simulink model "arduino"  (R2015b)
settings: Solver=VariableStepAuto  StartTime=0.0  StopTime=100.0  RelTol=1e-3
undefined symbols (not defined in the file or in its folder): serial
libraries: instrumentlib x3
settings Model: Creator=ovi  LastModifiedBy=ovi

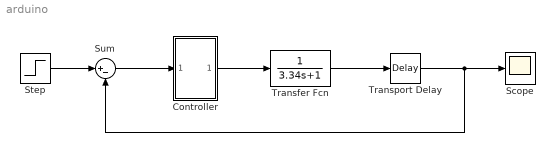
== system arduino ==
  "Controller " : Subsystem
  Scope : Scope
  Step : Step  SampleTime=0
  Sum : Sum  Inputs=|+-
  Transfer Fcn : TransferFcn  Denominator=[3.34 1]
  Transport Delay : TransportDelay  DelayTime=1.86
  wires:
  Sum/1 -> "Controller "/1(In1)
  "Controller "/1(Out1) -> Transfer Fcn/1
  Transfer Fcn/1 -> Transport Delay/1
  Transport Delay/1 -> Sum/2, Scope/1
  Step/1 -> Sum/1

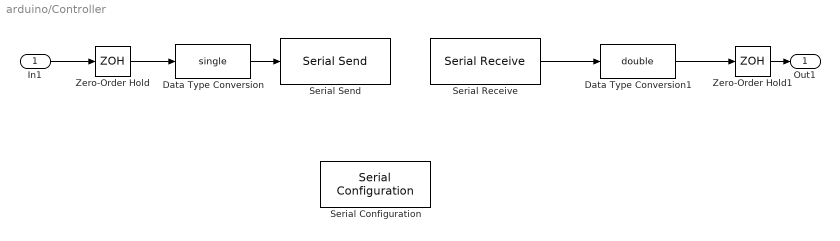
== system arduino/Controller  ==
  In1 : Inport
  Data Type Conversion : DataTypeConversion  OutDataTypeStr=single
  Data Type Conversion1 : DataTypeConversion  OutDataTypeStr=double
  Serial Configuration : instrumentlib/Serial Configuration  Priority=-200000  ComPortMenu=/dev/cu.usbmodem14101  ComPort=/dev/cu.usbmodem14101  ObjConstructor=serial('/dev/cu.usbmodem14101');  BaudRate=9600  DataBits=8  Parity=none  StopBits=1  FlowControl=none  Timeout=10  ByteOrder=LittleEndian
  Serial Receive : instrumentlib/Serial Receive  ComPortMenu=/dev/cu.usbmodem14101  ComPort=/dev/cu.usbmodem14101  ObjConstructor=serial('/dev/cu.usbmodem14101');  Terminator=<none>  DataSize=[1 1]  DataType=uint8  EnableBlockingMode=on  ActionDataUnavailable=Output last received value  CustomValue=0  SampleTime=0.1
  Serial Send : instrumentlib/Serial Send  ComPortMenu=/dev/cu.usbmodem14101  ComPort=/dev/cu.usbmodem14101  ObjConstructor=serial('/dev/cu.usbmodem14101');  Terminator=<none>  EnableBlockingMode=on
  Zero-Order Hold : ZeroOrderHold  SampleTime=0.1
  Zero-Order Hold1 : ZeroOrderHold  SampleTime=0.1
  Out1 : Outport
  wires:
  In1/1 -> Zero-Order Hold/1
  Zero-Order Hold1/1 -> Out1/1
  Data Type Conversion1/1 -> Zero-Order Hold1/1
  Data Type Conversion/1 -> Serial Send/1
  Zero-Order Hold/1 -> Data Type Conversion/1
  Serial Receive/1 -> Data Type Conversion1/1
